simulink model "AHRS_Sensor"  (R2019b)
settings: Solver=FixedStepDiscrete  StartTime=0.0  StopTime=10.0  FixedStep=0.01  MaxStep=0.001  RelTol=1e-6
model workspace (MAT data in the model file):
  A = [-0.0191  0.017  0.3839  -9.7924  -0.0008  -0.3371  0  0; 0.0136  -0.2994  0.0237  -0.5859  -0.0017  -0.0257  0.5374  0; 0.0405  -0.0026  -1.8394  0  0.0024  0.5281  0  -0.0015; 0  0  0.9985  0  0  0  0  0.0549; 0.001  -0.0017  -0.3381  0.0322  -0.0349  -0.4032  9.7777  0.1168; 0.013  0  -3.047  0  -0.229  -10.6199  0  -0.0333; 0  0  -0.0033  0  0  1  0  0.0598; 0.002  0.006  -0.5412  0  0.0039  -1.8554  0  -0.3487]
  B = [-10.3456  1.0793  0; -0.7293  0.0755  0; 27.09  -4.7239  -0.1857; 0  0  0; -1.082  -10.3713  4.7239; -27.2884  -156.4425  -1.069; 0  0  0; -4.8969  -27.9728  -12.9304]
  Cmeas = [0  0  0  1  0  0  0  0; 0  0  0  0  0  0  1  0; 0  0  0  0  0  0  0  1; 0  0  1  0  0  0  0  0; 0  0  0  0  0  1  0  0]
undefined symbols (not defined in the file or in its folder): p, phi, psi, q, r, theta, valid
settings Model: DataDictionary=HeliSystemDD.sldd  FPTRunName=Active  Creator=The MathWorks Inc.  LastModifiedBy=bpotter
settings DataIOCC: LimitDataPoints=on  SaveFormat=Array  SaveOutput=off  SaveTime=off  ReturnWorkspaceOutputs=off
settings OptimizationCC: BlockReduction=off  BooleanDataType=off  UseDivisionForNetSlopeComputation=on  LifeSpan=inf
settings DebuggingCC: SaveWithParameterizedLinksMsg=none  MergeDetectMultiDrivingBlocksExec=none  SignalResolutionControl=TryResolveAllWithWarning  AllowSymbolicDim=off  PregeneratedLibrarySubsystemCodeDiagnostic=none  StrictBusMsg=ErrorOnBusTreatedAsVector  NonBusSignalsTreatedAsBus=error  SFUnexpectedBacktrackingDiag=warning  SFNoUnconditionalDefaultTransitionDiag=warning  SFExecutionAtInitializationDiag=none  ArithmeticOperatorsInVariantConditions=warning
settings HardwareCC: ProdBitPerPointer=32  ProdBitPerSizeT=32  ProdBitPerPtrDiffT=32  ProdLargestAtomicFloat=None  ProdEndianess=Unspecified  ProdWordSize=32  ProdHWDeviceType=32-bit Generic  TargetUnknown=on
settings ModelReferenceCC: PropagateSignalLabelsOutOfModel=off
settings SFSimCC: SimUseLocalCustomCode=off  CustomCodeUndefinedFunction=UseInterfaceOnly
settings RTWCC: RTWUseLocalCustomCode=off
settings CodeAppCC: StateflowObjectComments=on
settings GRTTargetCC: TargetLangStandard=C89/C90 (ANSI)  GeneratePreprocessorConditionals=Disable all
settings ConfigComp: CovMetricSettings=dw  CovHtmlReporting=on  CovSaveCumulativeToWorkspaceVar=on  CovSaveSingleToWorkspaceVar=on  CovExternalEMLEnable=off

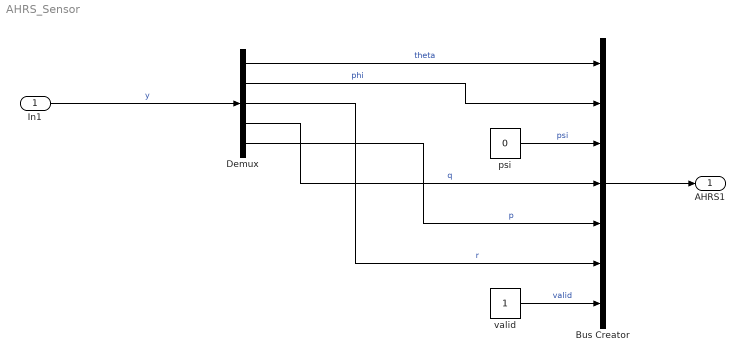
== system AHRS_Sensor ==
  In1 : Inport  OutDataTypeStr=double  PortDimensions=5
  Bus Creator : BusCreator  Inputs=theta,phi,psi,q,p,r,valid  OutDataTypeStr=Bus: AHRS_Bus  NonVirtualBus=on
  Demux : Demux  Outputs=5
  psi : Constant  Value=0  OutDataTypeStr=double  SampleTime=-1
  valid : Constant  OutDataTypeStr=boolean  SampleTime=-1
  AHRS1 : Outport  OutDataTypeStr=Bus: AHRS_Bus  PortDimensions=1  SampleTime=[0.01,0]  VectorParamsAs1DForOutWhenUnconnected=off  BusOutputAsStruct=on
  wires:
  In1/1 -> Demux/1  "y"
  valid/1 -> Bus Creator/7  "valid"
  Demux/1 -> Bus Creator/1  "theta"
  Demux/2 -> Bus Creator/2  "phi"
  psi/1 -> Bus Creator/3  "psi"
  Bus Creator/1 -> AHRS1/1
  Demux/3 -> Bus Creator/6  "r"
  Demux/5 -> Bus Creator/5  "p"
  Demux/4 -> Bus Creator/4  "q"
